simulink library "commutil2"  (Simulink 6.0)
undefined symbols (not defined in the file or in its folder): D, dBval, En, fuzz_val, IPValues, magnitude, OPValues, SatValue
libraries: dspsigattribs x12, dspsrcs4 x4, dspbuff3 x3, dspsigops x2, dspstat3 x2, dspmtrx3 x2, commutil2 x1, commblksprivate x1, simulink x1
settings Model: Creator=mmclerno  LastModifiedBy=mmclerno

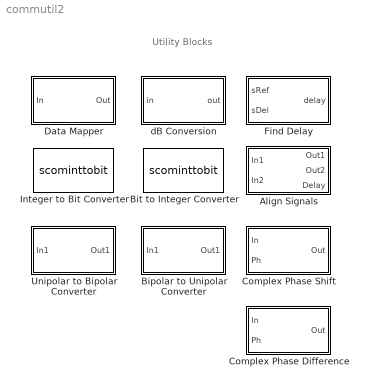
== system commutil2 ==
  note: Utility Blocks
  Align Signals : Subsystem  mask(Align Signals){corrLength=200, stopUpdate=off, numConstDelay=3}
      mask prompts: corrLength "Correlation window length (samples):"; stopUpdate "Disable recurring updates"; numConstDelay "Number of constant delay outputs to disable updates:"
      mask help: Align two signals s1 and s2 by finding the delay between them using cross-correlation techniques, then by delaying s1 by the computed delay. The input signal s2 should be delayed relative to the input s1, or else the computed delay will be incorrect, and the signals will not be properly aligned.
      mask init:
      | commblkalignsigs(gcb,'init');
      mask Help: helpview(commbhelp)
      mask CallbackString: |commblkalignsigs(gcb,'cbStopUpdate');|
      mask Display:
      | disp('Align\nSignals');
      | port_label('input', 1, 's1');
      | port_label('input', 2, 's2');
      | port_label('output', 1, 's1');
      | port_label('output', 2, 's2');
      | port_label('output', 3, 'delay');
  Bipolar to Unipolar Converter : Subsystem  mask(Bipolar to Unipolar Converter){M=4, polarity=Positive}
      mask prompts: M "M-ary number:"
      mask help: Convert a bipolar signal into a unipolar signal in the range [0, M-1], where M is the M-ary number.
      mask init:
      | if strcmp(polarity, 'Negative')
      |    pole = -1;
      | else
      |    pole = 1;
      | end
      mask Help: helpview(commbhelp);
      mask StyleString: edit,popup(Positive|Negative)
      mask Display: disp('Bipolar to\nUnipolar\nConverter');
  Bit to Integer Converter : S-Function  FunctionName=scominttobit  Parameters=nbits,1  mask(Bit to Integer Converter){nbits=3}
      mask prompts: nbits "Number of bits per integer:"
      mask help:
      | Map a vector of bits to a corresponding vector of integers. The first bit of the input vector is assumed to be the most significant bit (MSB). The Number of bits per integer value defines how many bits are mapped to each integer.
      |
      | In case of sample-based inputs, the input must be a vector whose width equals the number of bits per integer. In case of frame-based inputs, the input must be a column vector whose width is an integer multiple of the number of bits per integer.
      mask Help: helpview(commbhelp)
      mask Display: disp('Bit to Integer\nConverter')
  Complex Phase Difference : Subsystem
      mask Type: Complex Phase Difference
      mask Description: Output the phase difference between the two complex input signals. The range of the phase difference is from -pi to pi.
      mask Help: helpview(commbhelp)
      mask Display: disp('Complex Phase\nDifference');
  Complex Phase Shift : Subsystem
      mask Type: Complex Phase Shift
      mask Description: Shift the phase of the complex input signal by the "Ph" input value.
      mask Help: helpview(commbhelp)
      mask Display: disp('Complex\nPhase Shift');
  Data Mapper : Subsystem  mask(Data Mapper){MapMode=Binary to Gray, M=8, MapVec=[0 1 3 2 7 6 4 5]}
      mask prompts: MapMode "Mapping mode:"; M "Symbol set size (M):"; MapVec "Mapping vector:"
      mask help:
      | Map integer symbols from one coding scheme to another.
      |
      | The input can be either a scalar, a sample-based vector, or a frame-based column vector.
      mask init:
      | [En,IPValues,OPValues,SatValue]=commblkmapdata(gcb,'init',{MapMode M MapVec});
      mask Help: helpview(commbhelp)
      mask StyleString: popup(Binary to Gray|Gray to Binary|User Defined|Straight through),edit,edit
      mask CallbackString: commblkmapdata(gcb,'MapMode');||
      mask Display: disp('Data\nMapper');
  Find Delay : Subsystem  mask(Find Delay){corrLength=200, chgSigOP=off, stopUpdate=off, numConstDelay=3}
      mask prompts: corrLength "Correlation window length (samples):"; chgSigOP "Include "change signal" output port"; stopUpdate "Disable recurring updates"; numConstDelay "Number of constant delay outputs to disable updates:"
      mask help:
      | Find the delay between two signals sRef and sDel by finding the maximum of the cross-correlation function between them.  The signal sDel should be delayed relative to sRef, or else the computed delay will be incorrect.
      |
      | The optional "change signal" output port emits an impulse at the time instant when the current computed delay changes from the previous computed delay.
      mask init:
      | commblkfinddelay(gcb,'init');
      mask Help: helpview(commbhelp)
      mask CallbackString: |commblkfinddelay(gcb,'cbChgSigOP');|commblkfinddelay(gcb,'cbStopUpdate');|
      mask Display: disp('Find\nDelay');
  Integer to Bit Converter : S-Function  FunctionName=scominttobit  Parameters=nbits,2  mask(Integer to Bit Converter){nbits=3}
      mask prompts: nbits "Number of bits per integer:"
      mask help:
      | Map a vector of integers to a vector of bits. The first bit of the output vector is the most significant bit (MSB). The Number of bits per integer value defines how many bits are mapped from each integer.
      |
      | The input can be either a scalar or a frame-based column vector.
      mask Help: helpview(commbhelp)
      mask Display: disp('Integer to Bit\nConverter')
  Unipolar to Bipolar Converter : Subsystem  mask(Unipolar to Bipolar Converter){M=4, polarity=Positive}
      mask prompts: M "M-ary number:"
      mask help: Convert a unipolar signal in the range [0, M-1], where M is the M-ary number, into a bipolar signal.
      mask init:
      | if strcmp(polarity, 'Negative')
      |    pole = -1;
      | else
      |    pole = 1;
      | end
      mask Help: helpview(commbhelp);
      mask StyleString: edit,popup(Positive|Negative)
      mask Display: disp('Unipolar to\nBipolar\nConverter');
  dB Conversion : Subsystem  mask(dB Conversion){dBtype=dB, intype=Amplitude, R=1, fuzz=on}
      mask prompts: dBtype "Convert to:"; intype "Input signal:"; R "Load resistance (ohms):"; fuzz "Add  eps to input to protect against  "log(0) = -inf""
      mask help: Convert input of Watts or Volts to decibels. Voltage inputs are first converted to power relative to the specified load resistance, where P = (V^2)/R. When converting to dBm, the power is scaled to units of mWatts.
      mask init:
      | [str fuzz_val dBval] = dspblkdb2('init');
      | dspblkdb2('checkparam');
      | dspblkdb2('update');
      mask Help: web(dspbhelp);
      mask StyleString: popup(dB|dBm),popup(Power|Amplitude),edit,checkbox
      mask CallbackString: dspblkdb2|dspblkdb2||
      mask Display: disp(str)

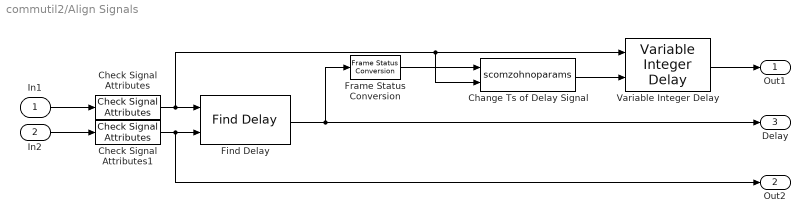
== system commutil2/Align Signals ==
  In1 : Inport
  In2 : Inport  Port=2
  Change Ts of Delay Signal : S-Function  FunctionName=scomzohnoparams
      mask Display:
      | disp('Zero Order\nHold');
      | port_label('input', 1, 'In');
      | port_label('input', 2, 'Ref');
      | port_label('output', 1, 'Out');
  Check Signal Attributes : dspsigattribs/Check Signal Attributes  SigAttribCheckMethod=Matches attributes exactly  Complexity=Ignore  Frame=Sample-based  DimsCheckMethod=Is...  Dimensions=Vector (1-D or 2-D)  DatatypeCheckMethod=Ignore  DatatypeGeneral=Boolean  DtypeFloatSpecific=Any floating-point  DtypeFixedSpecific=Any fixed-point  DtypeIntSpecific=Any integer  SampleMode=Ignore
  Check Signal Attributes1 : dspsigattribs/Check Signal Attributes  SigAttribCheckMethod=Matches attributes exactly  Complexity=Ignore  Frame=Sample-based  DimsCheckMethod=Is...  Dimensions=Vector (1-D or 2-D)  DatatypeCheckMethod=Ignore  DatatypeGeneral=Boolean  DtypeFloatSpecific=Any floating-point  DtypeFixedSpecific=Any fixed-point  DtypeIntSpecific=Any integer  SampleMode=Ignore
  Find Delay : commutil2/Find Delay  corrLength=corrLength  chgSigOP=off  stopUpdate=off  numConstDelay=3
  Frame Status Conversion : dspsigattribs/Frame Status Conversion  growRefPort=off  outframe=Frame-based
  Variable Integer Delay : dspsigops/Variable Integer Delay  dmax=corrLength  ic=0
  Out1 : Outport
  Out2 : Outport  Port=2
  Delay : Outport  Port=3
  wires:
  Frame Status Conversion/1 -> Change Ts of Delay Signal/1
  Find Delay/1 -> Frame Status Conversion/1, Delay/1
  Check Signal Attributes/1 -> Change Ts of Delay Signal/2, Variable Integer Delay/1, Find Delay/1
  Check Signal Attributes1/1 -> Out2/1, Find Delay/2
  Variable Integer Delay/1 -> Out1/1
  Change Ts of Delay Signal/1 -> Variable Integer Delay/2
  In1/1 -> Check Signal Attributes/1
  In2/1 -> Check Signal Attributes1/1

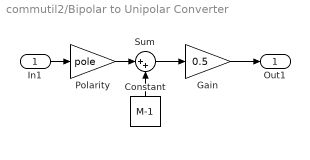
== system commutil2/Bipolar to Unipolar Converter ==
  In1 : Inport
  Constant : Constant  Orientation=up  Value=M-1
  Gain : Gain  Gain=0.5
  Polarity : Gain  Gain=pole
  Sum : Sum  Inputs=|++  InputSameDT=on
  Out1 : Outport
  wires:
  In1/1 -> Polarity/1
  Sum/1 -> Gain/1
  Constant/1 -> Sum/2
  Gain/1 -> Out1/1
  Polarity/1 -> Sum/1

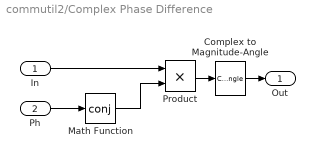
== system commutil2/Complex Phase Difference ==
  In : Inport
  Ph : Inport  Port=2
  Complex to Magnitude-Angle : ComplexToMagnitudeAngle  Output=Angle
  Math Function : Math  Operator=conj  SaturateOnIntegerOverflow=on
  Product : Product  SaturateOnIntegerOverflow=on  InputSameDT=on
  Out : Outport
  wires:
  Product/1 -> Complex to Magnitude-Angle/1
  Math Function/1 -> Product/2
  Ph/1 -> Math Function/1
  In/1 -> Product/1
  Complex to Magnitude-Angle/1 -> Out/1

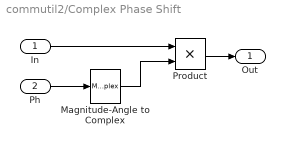
== system commutil2/Complex Phase Shift ==
  In : Inport
  Ph : Inport  Port=2
  Magnitude-Angle to Complex : MagnitudeAngleToComplex  Input=Angle  ConstantPart=1
  Product : Product  SaturateOnIntegerOverflow=on  InputSameDT=on
  Out : Outport
  wires:
  Product/1 -> Out/1
  Magnitude-Angle to Complex/1 -> Product/2
  Ph/1 -> Magnitude-Angle to Complex/1
  In/1 -> Product/1

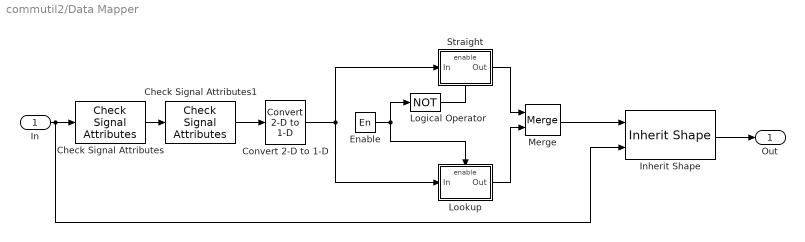
== system commutil2/Data Mapper ==
  In : Inport
  Check Signal Attributes : dspsigattribs/Check Signal Attributes  SigAttribCheckMethod=Matches attributes exactly  Complexity=Ignore  Frame=Ignore  DimsCheckMethod=Is...  Dimensions=Full matrix (2-D)  DatatypeCheckMethod=Ignore  DatatypeGeneral=Boolean  DtypeFloatSpecific=Any floating-point  DtypeFixedSpecific=Any fixed-point  DtypeIntSpecific=Any integer  SampleMode=Ignore
  Check Signal Attributes1 : dspsigattribs/Check Signal Attributes  SigAttribCheckMethod=Matches attributes exactly  Complexity=Ignore  Frame=Frame-based  DimsCheckMethod=Is...  Dimensions=Row vector (2-D)  DatatypeCheckMethod=Ignore  DatatypeGeneral=Boolean  DtypeFloatSpecific=Any floating-point  DtypeFixedSpecific=Any fixed-point  DtypeIntSpecific=Any integer  SampleMode=Ignore
  Convert 2-D to 1-D : dspsigattribs/Convert 2-D to 1-D
  Enable : Constant  Value=En
  Inherit Shape : commblksprivate/Inherit Shape
  Logical Operator : Logic  Operator=NOT  Inputs=1  OutDataTypeMode=Specify via dialog  LogicDataType=float('double')
  Lookup : Subsystem  TreatAsAtomicUnit=on
  Merge : Merge
  Straight : Subsystem  TreatAsAtomicUnit=on
  Out : Outport
  wires:
  Check Signal Attributes1/1 -> Convert 2-D to 1-D/1
  Check Signal Attributes/1 -> Check Signal Attributes1/1
  Inherit Shape/1 -> Out/1
  Merge/1 -> Inherit Shape/1
  Convert 2-D to 1-D/1 -> Lookup/1(In), Straight/1(In)
  Enable/1 -> Lookup/Enable, Logical Operator/1
  Logical Operator/1 -> Straight/Enable
  Lookup/1(Out) -> Merge/2
  In/1 -> Check Signal Attributes/1, Inherit Shape/2
  Straight/1(Out) -> Merge/1

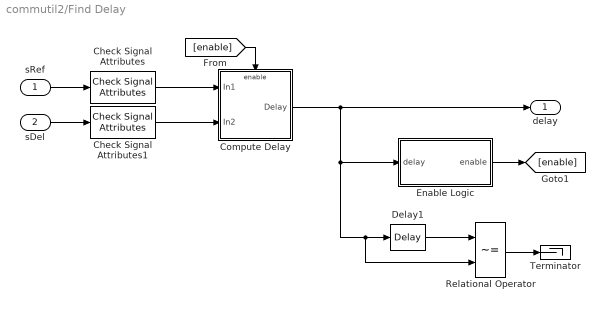
== system commutil2/Find Delay ==
  sRef : Inport
  sDel : Inport  Port=2
  Check Signal Attributes : dspsigattribs/Check Signal Attributes  SigAttribCheckMethod=Matches attributes exactly  Complexity=Ignore  Frame=Sample-based  DimsCheckMethod=Is...  Dimensions=Vector (1-D or 2-D)  DatatypeCheckMethod=Ignore  DatatypeGeneral=Boolean  DtypeFloatSpecific=Any floating-point  DtypeFixedSpecific=Any fixed-point  DtypeIntSpecific=Any integer  SampleMode=Ignore
  Check Signal Attributes1 : dspsigattribs/Check Signal Attributes  SigAttribCheckMethod=Matches attributes exactly  Complexity=Ignore  Frame=Sample-based  DimsCheckMethod=Is...  Dimensions=Vector (1-D or 2-D)  DatatypeCheckMethod=Ignore  DatatypeGeneral=Boolean  DtypeFloatSpecific=Any floating-point  DtypeFixedSpecific=Any fixed-point  DtypeIntSpecific=Any integer  SampleMode=Ignore
  Compute Delay : Subsystem
      mask Display: disp('Compute\nDelay')
  Delay1 : dspsigops/Delay  dly_unit=Samples  delay=1  ic_detail=off  dif_ic_for_ch=off  dif_ic_for_dly=off  ic=0  reset_popup=None
  Enable Logic : Subsystem
  Relational Operator : RelationalOperator  Operator=~=
  Terminator : Terminator
  delay : Outport
  wires:
  Check Signal Attributes/1 -> Compute Delay/1(In1)
  Enable Logic/1(enable) -> [enable]
  Check Signal Attributes1/1 -> Compute Delay/2(In2)
  [enable] -> Compute Delay/Enable
  sRef/1 -> Check Signal Attributes/1
  sDel/1 -> Check Signal Attributes1/1
  Delay1/1 -> Relational Operator/1
  Compute Delay/1(Delay) -> delay/1, Enable Logic/1(delay), Relational Operator/2, Delay1/1
  Relational Operator/1 -> Terminator/1

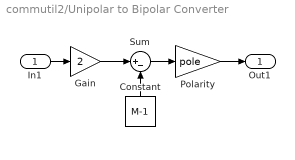
== system commutil2/Unipolar to Bipolar Converter ==
  In1 : Inport
  Constant : Constant  Orientation=up  Value=M-1
  Gain : Gain  Gain=2
  Polarity : Gain  Gain=pole
  Sum : Sum  Inputs=|+-  InputSameDT=on
  Out1 : Outport
  wires:
  Gain/1 -> Sum/1
  In1/1 -> Gain/1
  Sum/1 -> Polarity/1
  Constant/1 -> Sum/2
  Polarity/1 -> Out1/1

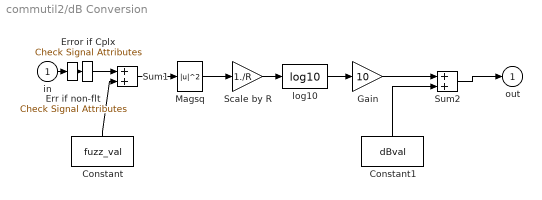
== system commutil2/dB Conversion ==
  in : Inport
  Constant : Constant  Orientation=up  Value=fuzz_val
  Constant1 : Constant  Orientation=up  Value=dBval
  Err if non-flt : dspsigattribs/Check Signal Attributes  SigAttribCheckMethod=Does not match attributes exactly  Complexity=Ignore  Frame=Ignore  DimsCheckMethod=Ignore  Dimensions=1-D  DatatypeCheckMethod=Is...  DatatypeGeneral=Floating-point  DtypeFloatSpecific=Any floating-point  DtypeFixedSpecific=Any fixed-point  DtypeIntSpecific=Any integer  SampleMode=Ignore
  Error if Cplx : dspsigattribs/Check Signal Attributes  SigAttribCheckMethod=Matches attributes exactly  Complexity=Complex  Frame=Ignore  DimsCheckMethod=Ignore  Dimensions=1-D  DatatypeCheckMethod=Ignore  DatatypeGeneral=Boolean  DtypeFloatSpecific=Any floating-point  DtypeFixedSpecific=Any fixed-point  DtypeIntSpecific=Any integer  SampleMode=Ignore
  Gain : Gain  Gain=10  SaturateOnIntegerOverflow=on
  Magsq : Math  Operator=magnitude^2  SaturateOnIntegerOverflow=on
  Scale by R : Gain  Gain=1./R  SaturateOnIntegerOverflow=on
  Sum1 : Sum  SaturateOnIntegerOverflow=on  InputSameDT=on
  Sum2 : Sum  SaturateOnIntegerOverflow=on  InputSameDT=on
  log10 : Math  Operator=log10  SaturateOnIntegerOverflow=on
  out : Outport  InitialOutput=0
  wires:
  log10/1 -> Gain/1
  Magsq/1 -> Scale by R/1
  Scale by R/1 -> log10/1
  Err if non-flt/1 -> Error if Cplx/1
  in/1 -> Err if non-flt/1
  Error if Cplx/1 -> Sum1/1
  Sum1/1 -> Magsq/1
  Constant/1 -> Sum1/2
  Gain/1 -> Sum2/1
  Sum2/1 -> out/1
  Constant1/1 -> Sum2/2

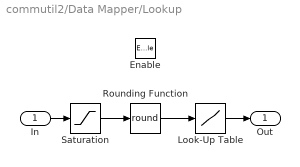
== system commutil2/Data Mapper/Lookup ==
  In : Inport
  Enable : EnablePort
  Look-Up Table : Lookup  InputValues=IPValues  OutputValues=OPValues  SaturateOnIntegerOverflow=on
  Rounding Function : Rounding  Operator=round
  Saturation : Saturate  UpperLimit=SatValue  LowerLimit=0
  Out : Outport
  wires:
  Rounding Function/1 -> Look-Up Table/1
  Saturation/1 -> Rounding Function/1
  Look-Up Table/1 -> Out/1
  In/1 -> Saturation/1

== system commutil2/Data Mapper/Straight ==
  In : Inport
  Enable : EnablePort
  Out : Outport
  wires:
  In/1 -> Out/1

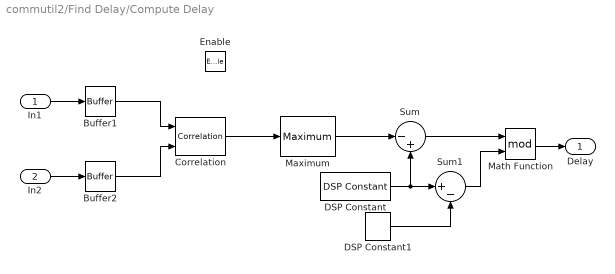
== system commutil2/Find Delay/Compute Delay ==
  In1 : Inport
  In2 : Inport  Port=2
  Enable : EnablePort
  Buffer1 : dspbuff3/Buffer  N=corrLength  V=0  ic=0
  Buffer2 : dspbuff3/Buffer  N=corrLength  V=0  ic=0
  Correlation : dspstat3/Correlation  domain=Time
  DSP Constant : dspsrcs4/DSP Constant  Value=corrLength  SampleMode=Discrete  discreteOutput=Sample-based  continuousOutput=Sample-based  sampTime=-1  framePeriod=2  dataType=Inherit from 'Constant value'  wordLen=16  udDataType=sfix(16)  fracBitsMode=Best precision  numFracBits=15  InterpretAs1D=-inf  Ts=-inf  FramebasedOutput=-inf
  DSP Constant1 : dspsrcs4/DSP Constant  Value=1  SampleMode=Discrete  discreteOutput=Sample-based  continuousOutput=Sample-based  sampTime=-1  framePeriod=2  dataType=Inherit from 'Constant value'  wordLen=16  udDataType=sfix(16)  fracBitsMode=Best precision  numFracBits=15  InterpretAs1D=-inf  Ts=-inf  FramebasedOutput=-inf
  Math Function : Math  Operator=mod  SaturateOnIntegerOverflow=on
  Maximum : dspstat3/Maximum  fcn=Index  reset=None
  Sum : Sum  Inputs=|-+  SaturateOnIntegerOverflow=on
  Sum1 : Sum  Inputs=|+-  SaturateOnIntegerOverflow=on
  Delay : Outport
  wires:
  Correlation/1 -> Maximum/1
  Buffer2/1 -> Correlation/2
  Buffer1/1 -> Correlation/1
  In1/1 -> Buffer1/1
  In2/1 -> Buffer2/1
  Maximum/1 -> Sum/1
  DSP Constant/1 -> Sum/2, Sum1/1
  DSP Constant1/1 -> Sum1/2
  Sum/1 -> Math Function/1
  Sum1/1 -> Math Function/2
  Math Function/1 -> Delay/1

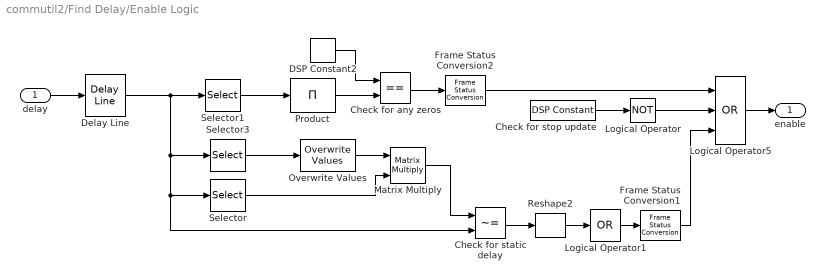
== system commutil2/Find Delay/Enable Logic ==
  delay : Inport
  Check for any zeros : RelationalOperator  Operator===
  Check for static delay : RelationalOperator  Operator=~=
  Check for stop update : dspsrcs4/DSP Constant  Value=stopUpdate  SampleMode=Discrete  discreteOutput=Sample-based  continuousOutput=Sample-based  sampTime=-1  framePeriod=2  dataType=boolean  wordLen=16  udDataType=sfix(16)  fracBitsMode=Best precision  numFracBits=15  InterpretAs1D=-inf  Ts=-inf  FramebasedOutput=-inf
      settings: additionalParams=on
  DSP Constant2 : dspsrcs4/DSP Constant  Value=0  SampleMode=Discrete  discreteOutput=Frame-based  continuousOutput=Sample-based  sampTime=-1  framePeriod=-1  dataType=Inherit from 'Constant value'  wordLen=16  udDataType=sfix(16)  fracBitsMode=Best precision  numFracBits=15  InterpretAs1D=-inf  Ts=-inf  FramebasedOutput=-inf
  Delay Line : dspbuff3/Delay Line  siz=numConstDelay  ic=0
  Frame Status Conversion1 : dspsigattribs/Frame Status Conversion  growRefPort=off  outframe=Sample-based
  Frame Status Conversion2 : dspsigattribs/Frame Status Conversion  growRefPort=off  outframe=Sample-based
  Logical Operator : Logic  Operator=NOT  AllPortsSameDT=off
  Logical Operator1 : Logic  Operator=OR  Inputs=1  AllPortsSameDT=off
  Logical Operator5 : Logic  Operator=OR  Inputs=3
  Matrix Multiply : dspmtrx3/Matrix Multiply  numInputPorts=2  OptimizationLevel=None
  Overwrite Values : dspmtrx3/Overwrite Values  OverWriteDiag=Submatrix  valFrom2ndIP=Specify via dialog  ConstValue=1  RowSpan=All rows  RowStartMode=Index  RowStartIndex=2  RowEndMode=Last  RowEndIndex=1  ColSpan=One column  ColStartMode=First  ColStartIndex=1  ColEndMode=Last  ColEndIndex=1  DiagSpan=Range of elements  DiagStartMode=Index  DiagStartIndex=2  DiagEndMode=Index  DiagEndIndex=4
  Product : Product  Inputs=1  OutDataTypeMode=double  SaturateOnIntegerOverflow=on
  Reshape2 : simulink/Math Operations/Reshape  OutputDimensionality=Column vector  OutputDimensions=[1,1]
  Selector : Selector  InputType=Matrix  Elements=[1]  Columns=-1  InputPortWidth=numConstDelay
  Selector1 : Selector  InputType=Matrix  Elements=[1]  Rows=-1  InputPortWidth=numConstDelay
  Selector3 : Selector  InputType=Matrix  Elements=[1]  Rows=-1  InputPortWidth=numConstDelay
  enable : Outport
  wires:
  Check for static delay/1 -> Reshape2/1
  Reshape2/1 -> Logical Operator1/1
  Matrix Multiply/1 -> Check for static delay/1
  Selector/1 -> Matrix Multiply/2
  Overwrite Values/1 -> Matrix Multiply/1
  Selector3/1 -> Overwrite Values/1
  Selector1/1 -> Product/1
  delay/1 -> Delay Line/1
  Delay Line/1 -> Selector1/1, Selector3/1, Check for static delay/2, Selector/1
  Check for stop update/1 -> Logical Operator/1
  Logical Operator/1 -> Logical Operator5/2
  Frame Status Conversion1/1 -> Logical Operator5/3
  Logical Operator1/1 -> Frame Status Conversion1/1
  Product/1 -> Check for any zeros/2
  DSP Constant2/1 -> Check for any zeros/1
  Check for any zeros/1 -> Frame Status Conversion2/1
  Frame Status Conversion2/1 -> Logical Operator5/1
  Logical Operator5/1 -> enable/1
